simulink model "Spange_Thrust_simulation_4mode"  (R2016a)
settings: Solver=ode3  StartTime=0.0  StopTime=4  RelTol=1e-3
values from neighbouring files (symbols this model uses):
  C = [C1;C2;C3]    [Spange_init.m]
  D = 3.0/100    (= 0.03)    [Spange_init.m]
  eps_c = 5    [Spange_init.m]
  epsilon = 0.5    [Spange_init.m]
  hd = c2d(H1,0.1,'foh')    [Spange_init.m]
  hd2 = c2d(H2,0.01,'zoh')    [Spange_init.m]
  I_s = 0.05    [Spange_init.m]
  k_cc = 1    [Spange_init.m]
  K_omega = 0.3    [Spange_init.m]
  K_q1f = 0.0113    [Spange_init.m]
  K_q1r = K_q1f    (= 0.0113)    [Spange_init.m]
  K_q2f = 0.0117    [Spange_init.m]
  K_q2r = K_q2f    (= 0.0117)    [Spange_init.m]
  K_q3f = 0.0113    [Spange_init.m]
  K_q3r = K_q3f    (= 0.0113)    [Spange_init.m]
  K_T1f = 0.3763    [Spange_init.m]
  K_T1r = K_T1f    (= 0.3763)    [Spange_init.m]
  K_T2f = 0.3901    [Spange_init.m]
  K_T2r = K_T2f    (= 0.3901)    [Spange_init.m]
  K_T3f = 0.3776    [Spange_init.m]
  K_T3r = K_T3f    (= 0.3776)    [Spange_init.m]
  Kp = 0.3    [Spange_init.m]
  Max_Acceleration = 2    [Spange_init.m]
  Max_rotation = 12*sqrt(lambda)    [Spange_init.m]
  Max_thrust = 1.5034    [Spange_init.m]
  Min_thrust = -0.85    [Spange_init.m]
  mode = 4    [Spange_init.m]
  n_c = 5    [Spange_init.m]
  n_max = 64.6    [Spange_init.m]
  p_cc = 0.5    [Spange_init.m]
  Q_f0 = 0.3    [Spange_init.m]
  r_cc = 4    [Spange_init.m]
  Rho = Rho_m    (= 1000)    [Spange_init.m]
  td = [1;0;0]    [Spange_init.m]
  Thruster_control = 1    [Spange_init.m]
  ThrusterPosX = [Thruster.T1(1) Thruster.T2(1) Thruster.T3(1)]    [Spange_init.m]
  ThrusterPosY = [Thruster.T1(2) Thruster.T2(2) Thruster.T3(2)]    [Spange_init.m]
  u_e = [1 0 1 0 0 ... (first row only)    [Spange_init.m]
undefined symbols (not defined in the file or in its folder): Thruster
libraries: simulink_extras x16, simulink x8
(part 2 of 3)

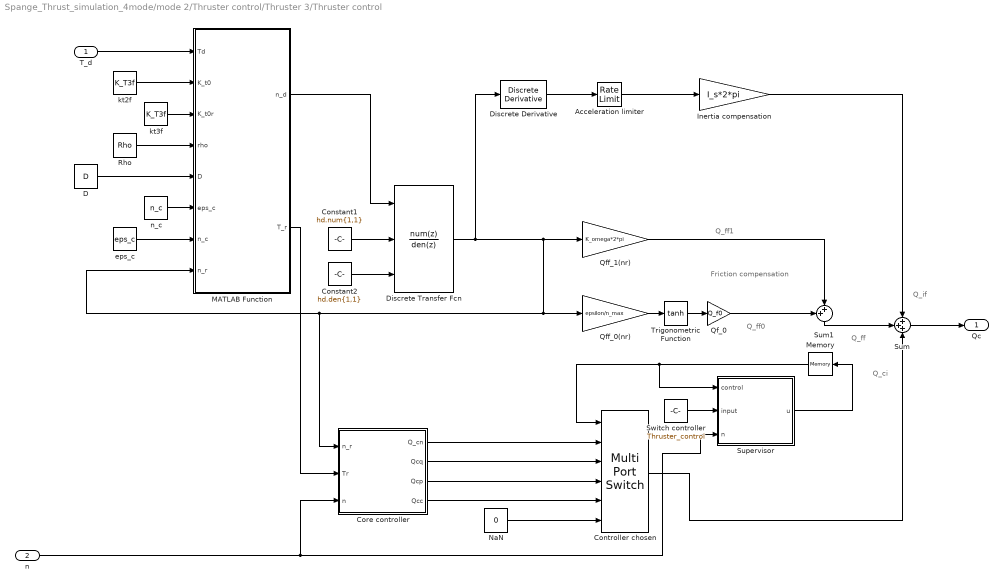
== system Spange_Thrust_simulation_4mode/mode 2/Thruster control/Thruster 3/Thruster control ==
  note: Friction compensation
  note: Q_ff1
  note: Q_ff0
  note: Q_ff
  note: Q_if
  note: Q_ci
  "T_d " : Inport
  n : Inport  Port=2
  Acceleration limiter : RateLimiter  RisingSlewLimit=Max_Acceleration  FallingSlewLimit=-Max_Acceleration  SampleTimeMode=inherited
  Constant1 : Constant  Value=hd.num{1,1}  VectorParams1D=off
  Constant2 : Constant  Value=hd.den{1,1}  VectorParams1D=off
  Controller chosen : MultiPortSwitch  Inputs=5
  Core controller : Subsystem
  D : Constant  Value=D  VectorParams1D=off
  Discrete Transfer Fcn : DiscreteTransferFcn  NumeratorSource=Input port  Numerator=[8.76e-05 0.0003481 8.648e-05]  DenominatorSource=Input port  Denominator=[1 -1.974 0.9746]  SampleTime=0.01  a0EqualsOne=on
      settings: InputPortMap=u0,p1,p3
  Discrete Derivative : simulink/Discrete/Discrete Derivative  gainval=1.0  ICPrevScaledInput=0.0  InputProcessing=Inherited  OutMin=[]  OutMax=[]  OutDataType=fixdt(1, 16)  OutScaling=2^-10  DoSatur=off
  Inertia compensation : Gain  Gain=I_s*2*pi
  MATLAB Function : MATLAB Function  TreatAsAtomicUnit=on
  Memory : Memory  X0=1
  NaN : Constant  Value=0
  Qf_0 : Gain  Gain=Q_f0
  Qff_0(nr) : Gain  Gain=epsilon/n_max
  Qff_1(nr) : Gain  Gain=K_omega*2*pi
  Rho : Constant  Value=Rho  VectorParams1D=off
  Sum : Sum  Inputs=+++
  Sum1 : Sum  Inputs=++|
  Supervisor : MATLAB Function  TreatAsAtomicUnit=on
  Switch controller : Constant  Value=Thruster_control
  Trigonometric Function : Trigonometry  Operator=tanh
  eps_c : Constant  Value=eps_c  VectorParams1D=off
  kt2f : Constant  Value=K_T3f  VectorParams1D=off
  kt3f : Constant  Value=K_T3f  VectorParams1D=off
  n_c : Constant  Value=n_c  VectorParams1D=off
  Qc : Outport
  wires:
  kt3f/1 -> MATLAB Function/3(K_t0r)
  kt2f/1 -> MATLAB Function/2(K_t0)
  Sum/1 -> Qc/1
  Discrete Transfer Fcn/1 -> Qff_1(nr)/1, Qff_0(nr)/1, Core controller/1(n_r), MATLAB Function/8(n_r), Discrete Derivative/1
  Acceleration limiter/1 -> Inertia compensation/1
  n/1 -> Supervisor/3(n), Core controller/3("n ")
  MATLAB Function/1(n_d) -> Discrete Transfer Fcn/1
  Constant2/1 -> Discrete Transfer Fcn/3
  Constant1/1 -> Discrete Transfer Fcn/2
  eps_c/1 -> MATLAB Function/7(n_c)
  n_c/1 -> MATLAB Function/6(eps_c)
  D/1 -> MATLAB Function/5(D)
  Rho/1 -> MATLAB Function/4(rho)
  "T_d "/1 -> MATLAB Function/1(Td)
  Switch controller/1 -> Supervisor/2(input)
  Core controller/2(Qcq) -> Controller chosen/3
  Core controller/3(Qcp) -> Controller chosen/4
  Inertia compensation/1 -> Sum/1
  Controller chosen/1 -> Sum/3
  Qf_0/1 -> Sum1/1
  Qff_1(nr)/1 -> Sum1/2
  Memory/1 -> Controller chosen/1, Supervisor/1(control)
  Supervisor/1(u) -> Memory/1
  NaN/1 -> Controller chosen/6
  Core controller/4(Qcc) -> Controller chosen/5
  Core controller/1(Q_cn) -> Controller chosen/2
  Sum1/1 -> Sum/2
  Trigonometric Function/1 -> Qf_0/1
  Qff_0(nr)/1 -> Trigonometric Function/1
  Discrete Derivative/1 -> Acceleration limiter/1
  MATLAB Function/2(T_r) -> Core controller/2("Tr ")

== system Spange_Thrust_simulation_4mode/mode 3/Thruster control/Thruster 1/Propeller Hydrodynamics ==
  env : Inport
  n : Inport  Port=2
  Actual Force and Torque : MATLAB Function  TreatAsAtomicUnit=on
  D1 : Constant  Value=D
  Kq1 : Constant  Value=K_q1f
  Kqr1 : Constant  Value=K_q1r
  Ktf : Constant  Value=K_T1f
  Ktr : Constant  Value=K_T1r
  Rho1 : Constant  Value=Rho
  eps_c1 : Constant  Value=eps_c
  Ta : Outport
  Qa : Outport  Port=2
  wires:
  eps_c1/1 -> Actual Force and Torque/8(eps_c)
  Kqr1/1 -> Actual Force and Torque/5(Kqr)
  Ktr/1 -> Actual Force and Torque/4(Ktr)
  Actual Force and Torque/1(Ta) -> Ta/1
  Ktf/1 -> Actual Force and Torque/3(Kt)
  env/1 -> Actual Force and Torque/9(env)
  Rho1/1 -> Actual Force and Torque/6(Rho)
  Actual Force and Torque/2(Qa) -> Qa/1
  Kq1/1 -> Actual Force and Torque/2(Kq)
  D1/1 -> Actual Force and Torque/7(D)
  n/1 -> Actual Force and Torque/1(n)

== system Spange_Thrust_simulation_4mode/mode 3/Thruster control/Thruster 1/Shaft dynamics ==
  Qm : Inport
  Qa : Inport  Port=2
  Constant : Constant  Value=0
  Finding rotation speed : Gain  Gain=1/(2*pi*I_s)
  Integrator : Integrator  ExternalReset=either
  K_omega : Gain  Gain=K_omega*2*pi
  Sum : Sum  Inputs=-+-
  n : Outport
  wires:
  Constant/1 -> Integrator/2
  Integrator/1 -> K_omega/1, n/1
  Finding rotation speed/1 -> Integrator/1
  K_omega/1 -> Sum/3
  Qa/1 -> Sum/1
  Sum/1 -> Finding rotation speed/1
  Qm/1 -> Sum/2

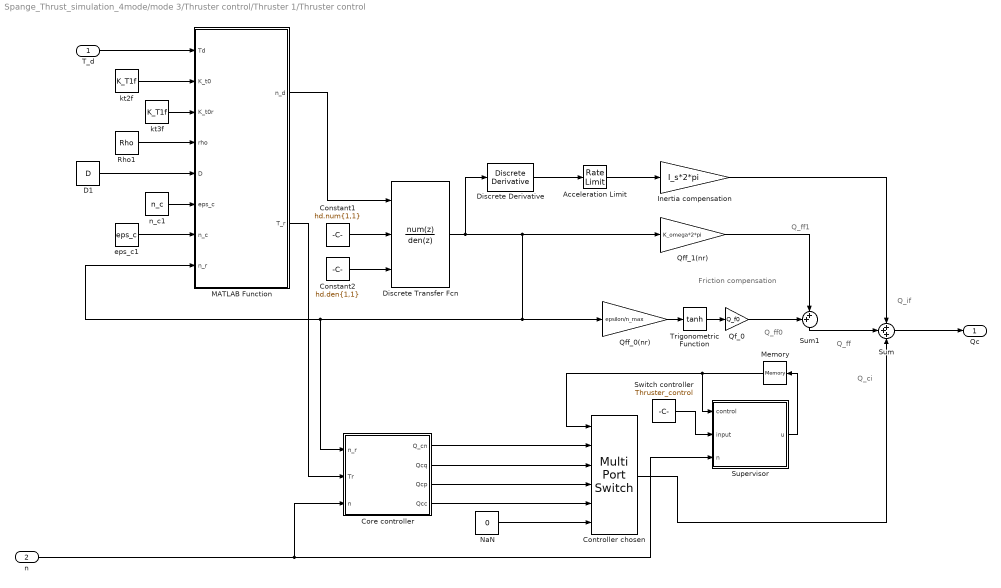
== system Spange_Thrust_simulation_4mode/mode 3/Thruster control/Thruster 1/Thruster control ==
  note: Friction compensation
  note: Q_ff1
  note: Q_ff0
  note: Q_ff
  note: Q_if
  note: Q_ci
  "T_d " : Inport
  n : Inport  Port=2
  Acceleration Limit : RateLimiter  RisingSlewLimit=Max_Acceleration  FallingSlewLimit=-Max_Acceleration  SampleTimeMode=inherited
  Constant1 : Constant  Value=hd.num{1,1}  VectorParams1D=off
  Constant2 : Constant  Value=hd.den{1,1}  VectorParams1D=off
  Controller chosen : MultiPortSwitch  Inputs=5
  Core controller : Subsystem
  D1 : Constant  Value=D  VectorParams1D=off
  Discrete Transfer Fcn : DiscreteTransferFcn  NumeratorSource=Input port  Numerator=[8.76e-05 0.0003481 8.648e-05]  DenominatorSource=Input port  Denominator=[1 -1.974 0.9746]  SampleTime=0.01  a0EqualsOne=on
      settings: InputPortMap=u0,p1,p3
  Discrete Derivative : simulink/Discrete/Discrete Derivative  gainval=1.0  ICPrevScaledInput=0.0  InputProcessing=Inherited  OutMin=[]  OutMax=[]  OutDataType=fixdt(1, 16)  OutScaling=2^-10  DoSatur=off
  Inertia compensation : Gain  Gain=I_s*2*pi
  MATLAB Function : MATLAB Function  TreatAsAtomicUnit=on
  Memory : Memory  X0=1  InheritSampleTime=on
  NaN : Constant  Value=0
  Qf_0 : Gain  Gain=Q_f0
  Qff_0(nr) : Gain  Gain=epsilon/n_max
  Qff_1(nr) : Gain  Gain=K_omega*2*pi
  Rho1 : Constant  Value=Rho  VectorParams1D=off
  Sum : Sum  Inputs=+++
  Sum1 : Sum  Inputs=++|
  Supervisor : MATLAB Function  TreatAsAtomicUnit=on
  Switch controller : Constant  Value=Thruster_control
  Trigonometric Function : Trigonometry  Operator=tanh
  eps_c1 : Constant  Value=eps_c  VectorParams1D=off
  kt2f : Constant  Value=K_T1f  VectorParams1D=off
  kt3f : Constant  Value=K_T1f  VectorParams1D=off
  n_c1 : Constant  Value=n_c  VectorParams1D=off
  Qc : Outport
  wires:
  Sum/1 -> Qc/1
  "T_d "/1 -> MATLAB Function/1(Td)
  Discrete Transfer Fcn/1 -> Discrete Derivative/1, Qff_1(nr)/1, Qff_0(nr)/1, MATLAB Function/8(n_r), Core controller/1(n_r)
  Acceleration Limit/1 -> Inertia compensation/1
  n/1 -> Supervisor/3(n), Core controller/3("n ")
  Inertia compensation/1 -> Sum/1
  Constant2/1 -> Discrete Transfer Fcn/3
  Constant1/1 -> Discrete Transfer Fcn/2
  Sum1/1 -> Sum/2
  Discrete Derivative/1 -> Acceleration Limit/1
  Core controller/1(Q_cn) -> Controller chosen/2
  Core controller/4(Qcc) -> Controller chosen/5
  Core controller/3(Qcp) -> Controller chosen/4
  Core controller/2(Qcq) -> Controller chosen/3
  Controller chosen/1 -> Sum/3
  Switch controller/1 -> Supervisor/2(input)
  Qf_0/1 -> Sum1/1
  Qff_1(nr)/1 -> Sum1/2
  Memory/1 -> Supervisor/1(control), Controller chosen/1
  Supervisor/1(u) -> Memory/1
  NaN/1 -> Controller chosen/6
  Trigonometric Function/1 -> Qf_0/1
  Qff_0(nr)/1 -> Trigonometric Function/1
  MATLAB Function/1(n_d) -> Discrete Transfer Fcn/1
  MATLAB Function/2(T_r) -> Core controller/2("Tr ")
  kt2f/1 -> MATLAB Function/2(K_t0)
  eps_c1/1 -> MATLAB Function/7(n_c)
  D1/1 -> MATLAB Function/5(D)
  Rho1/1 -> MATLAB Function/4(rho)
  kt3f/1 -> MATLAB Function/3(K_t0r)
  n_c1/1 -> MATLAB Function/6(eps_c)

== system Spange_Thrust_simulation_4mode/mode 3/Thruster control/Thruster 2/Propeller Hydrodynamics ==
  env : Inport
  n : Inport  Port=2
  Actual Force and Torque : MATLAB Function  TreatAsAtomicUnit=on
  D1 : Constant  Value=D
  Kq1 : Constant  Value=K_q2f
  Kqr1 : Constant  Value=K_q2r
  Ktf : Constant  Value=K_T2f
  Ktr : Constant  Value=K_T2r
  Rho1 : Constant  Value=Rho
  eps_c1 : Constant  Value=eps_c
  Ta : Outport
  Qa : Outport  Port=2
  wires:
  eps_c1/1 -> Actual Force and Torque/8(eps_c)
  Kqr1/1 -> Actual Force and Torque/5(Kqr)
  Ktr/1 -> Actual Force and Torque/4(Ktr)
  Actual Force and Torque/1(Ta) -> Ta/1
  Ktf/1 -> Actual Force and Torque/3(Kt)
  env/1 -> Actual Force and Torque/9(env)
  Rho1/1 -> Actual Force and Torque/6(Rho)
  Actual Force and Torque/2(Qa) -> Qa/1
  Kq1/1 -> Actual Force and Torque/2(Kq)
  D1/1 -> Actual Force and Torque/7(D)
  n/1 -> Actual Force and Torque/1(n)

== system Spange_Thrust_simulation_4mode/mode 3/Thruster control/Thruster 2/Shaft dynamics ==
  Qm : Inport
  Qa : Inport  Port=2
  Constant : Constant  Value=0
  Finding rotation speed : Gain  Gain=1/(2*pi*I_s)
  Integrator : Integrator  ExternalReset=either
  K_omega : Gain  Gain=K_omega*2*pi
  Sum : Sum  Inputs=-+-
  n : Outport
  wires:
  Constant/1 -> Integrator/2
  Integrator/1 -> n/1, K_omega/1
  Finding rotation speed/1 -> Integrator/1
  K_omega/1 -> Sum/3
  Qa/1 -> Sum/1
  Sum/1 -> Finding rotation speed/1
  Qm/1 -> Sum/2

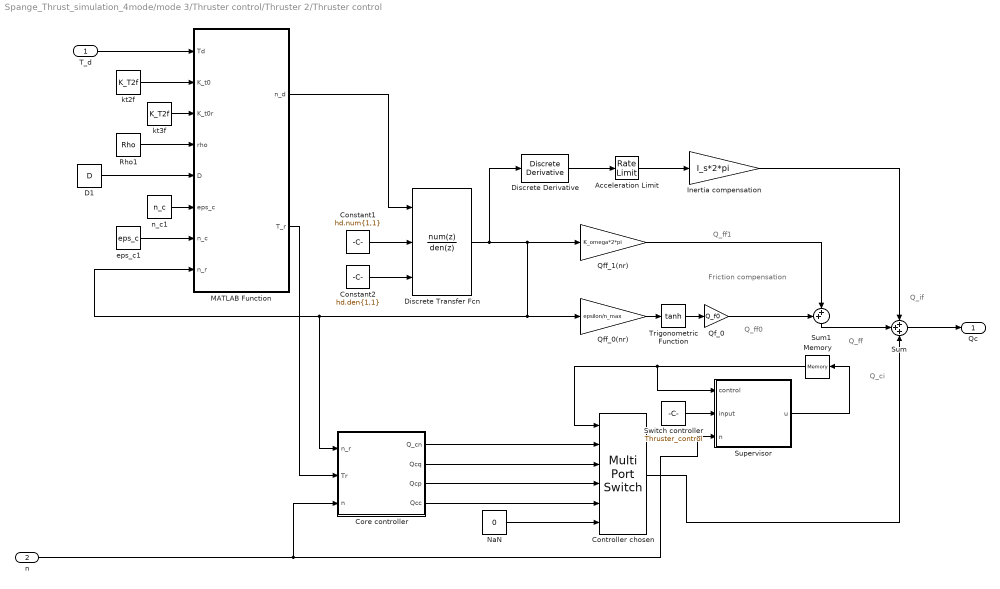
== system Spange_Thrust_simulation_4mode/mode 3/Thruster control/Thruster 2/Thruster control ==
  note: Friction compensation
  note: Q_ff1
  note: Q_ff0
  note: Q_ff
  note: Q_if
  note: Q_ci
  "T_d " : Inport
  n : Inport  Port=2
  Acceleration Limit : RateLimiter  RisingSlewLimit=Max_Acceleration  FallingSlewLimit=-Max_Acceleration  SampleTimeMode=inherited
  Constant1 : Constant  Value=hd.num{1,1}  VectorParams1D=off
  Constant2 : Constant  Value=hd.den{1,1}  VectorParams1D=off
  Controller chosen : MultiPortSwitch  Inputs=5
  Core controller : Subsystem
  D1 : Constant  Value=D  VectorParams1D=off
  Discrete Transfer Fcn : DiscreteTransferFcn  NumeratorSource=Input port  Numerator=[8.76e-05 0.0003481 8.648e-05]  DenominatorSource=Input port  Denominator=[1 -1.974 0.9746]  SampleTime=0.01  a0EqualsOne=on
      settings: InputPortMap=u0,p1,p3
  Discrete Derivative : simulink/Discrete/Discrete Derivative  gainval=1.0  ICPrevScaledInput=0.0  InputProcessing=Inherited  OutMin=[]  OutMax=[]  OutDataType=fixdt(1, 16)  OutScaling=2^-10  DoSatur=off
  Inertia compensation : Gain  Gain=I_s*2*pi
  MATLAB Function : MATLAB Function  TreatAsAtomicUnit=on
  Memory : Memory  X0=1
  NaN : Constant  Value=0
  Qf_0 : Gain  Gain=Q_f0
  Qff_0(nr) : Gain  Gain=epsilon/n_max
  Qff_1(nr) : Gain  Gain=K_omega*2*pi
  Rho1 : Constant  Value=Rho  VectorParams1D=off
  Sum : Sum  Inputs=+++
  Sum1 : Sum  Inputs=++|
  Supervisor : MATLAB Function  TreatAsAtomicUnit=on
  Switch controller : Constant  Value=Thruster_control
  Trigonometric Function : Trigonometry  Operator=tanh
  eps_c1 : Constant  Value=eps_c  VectorParams1D=off
  kt2f : Constant  Value=K_T2f  VectorParams1D=off
  kt3f : Constant  Value=K_T2f  VectorParams1D=off
  n_c1 : Constant  Value=n_c  VectorParams1D=off
  Qc : Outport
  wires:
  Sum/1 -> Qc/1
  Discrete Transfer Fcn/1 -> Qff_1(nr)/1, Core controller/1(n_r), MATLAB Function/8(n_r), Qff_0(nr)/1, Discrete Derivative/1
  Acceleration Limit/1 -> Inertia compensation/1
  n/1 -> Supervisor/3(n), Core controller/3("n ")
  Discrete Derivative/1 -> Acceleration Limit/1
  MATLAB Function/1(n_d) -> Discrete Transfer Fcn/1
  Constant2/1 -> Discrete Transfer Fcn/3
  Constant1/1 -> Discrete Transfer Fcn/2
  "T_d "/1 -> MATLAB Function/1(Td)
  Switch controller/1 -> Supervisor/2(input)
  Core controller/2(Qcq) -> Controller chosen/3
  Core controller/3(Qcp) -> Controller chosen/4
  Inertia compensation/1 -> Sum/1
  Controller chosen/1 -> Sum/3
  Qf_0/1 -> Sum1/1
  Qff_1(nr)/1 -> Sum1/2
  Memory/1 -> Controller chosen/1, Supervisor/1(control)
  Supervisor/1(u) -> Memory/1
  NaN/1 -> Controller chosen/6
  Core controller/4(Qcc) -> Controller chosen/5
  Core controller/1(Q_cn) -> Controller chosen/2
  Sum1/1 -> Sum/2
  Trigonometric Function/1 -> Qf_0/1
  Qff_0(nr)/1 -> Trigonometric Function/1
  MATLAB Function/2(T_r) -> Core controller/2("Tr ")
  kt2f/1 -> MATLAB Function/2(K_t0)
  eps_c1/1 -> MATLAB Function/7(n_c)
  D1/1 -> MATLAB Function/5(D)
  Rho1/1 -> MATLAB Function/4(rho)
  kt3f/1 -> MATLAB Function/3(K_t0r)
  n_c1/1 -> MATLAB Function/6(eps_c)

== system Spange_Thrust_simulation_4mode/mode 4/Thruster control/Thruster 1/Propeller Hydrodynamics ==
  env : Inport
  n : Inport  Port=2
  Actual Force and Torque : MATLAB Function  TreatAsAtomicUnit=on
  D1 : Constant  Value=D
  Kq1 : Constant  Value=K_q1f
  Kqr1 : Constant  Value=K_q1r
  Ktf : Constant  Value=K_T1f
  Ktr : Constant  Value=K_T1r
  Rho1 : Constant  Value=Rho
  eps_c1 : Constant  Value=eps_c
  Ta : Outport
  Qa : Outport  Port=2
  wires:
  eps_c1/1 -> Actual Force and Torque/8(eps_c)
  Kqr1/1 -> Actual Force and Torque/5(Kqr)
  Ktr/1 -> Actual Force and Torque/4(Ktr)
  Actual Force and Torque/1(Ta) -> Ta/1
  Ktf/1 -> Actual Force and Torque/3(Kt)
  env/1 -> Actual Force and Torque/9(env)
  Rho1/1 -> Actual Force and Torque/6(Rho)
  Actual Force and Torque/2(Qa) -> Qa/1
  Kq1/1 -> Actual Force and Torque/2(Kq)
  D1/1 -> Actual Force and Torque/7(D)
  n/1 -> Actual Force and Torque/1(n)

== system Spange_Thrust_simulation_4mode/mode 4/Thruster control/Thruster 1/Shaft dynamics ==
  Qm : Inport
  Qa : Inport  Port=2
  Constant : Constant  Value=0
  Finding rotation speed : Gain  Gain=1/(2*pi*I_s)
  Integrator : Integrator  ExternalReset=either
  K_omega : Gain  Gain=K_omega*2*pi
  Sum : Sum  Inputs=-+-
  n : Outport
  wires:
  Constant/1 -> Integrator/2
  Integrator/1 -> K_omega/1, n/1
  Finding rotation speed/1 -> Integrator/1
  K_omega/1 -> Sum/3
  Qa/1 -> Sum/1
  Sum/1 -> Finding rotation speed/1
  Qm/1 -> Sum/2

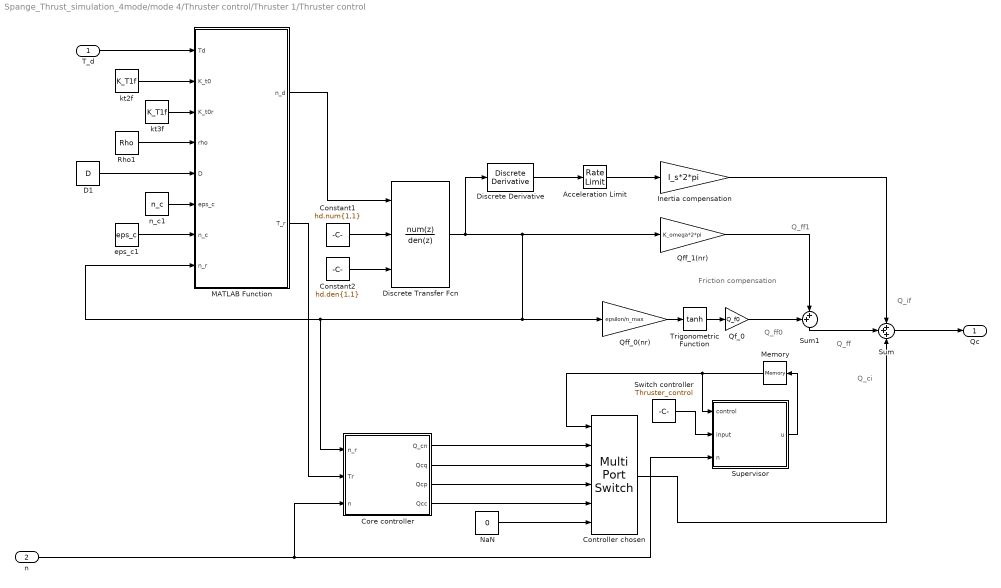
== system Spange_Thrust_simulation_4mode/mode 4/Thruster control/Thruster 1/Thruster control ==
  note: Friction compensation
  note: Q_ff1
  note: Q_ff0
  note: Q_ff
  note: Q_if
  note: Q_ci
  "T_d " : Inport
  n : Inport  Port=2
  Acceleration Limit : RateLimiter  RisingSlewLimit=Max_Acceleration  FallingSlewLimit=-Max_Acceleration  SampleTimeMode=inherited
  Constant1 : Constant  Value=hd.num{1,1}  VectorParams1D=off
  Constant2 : Constant  Value=hd.den{1,1}  VectorParams1D=off
  Controller chosen : MultiPortSwitch  Inputs=5
  Core controller : Subsystem
  D1 : Constant  Value=D  VectorParams1D=off
  Discrete Transfer Fcn : DiscreteTransferFcn  NumeratorSource=Input port  Numerator=[8.76e-05 0.0003481 8.648e-05]  DenominatorSource=Input port  Denominator=[1 -1.974 0.9746]  SampleTime=0.01  a0EqualsOne=on
      settings: InputPortMap=u0,p1,p3
  Discrete Derivative : simulink/Discrete/Discrete Derivative  gainval=1.0  ICPrevScaledInput=0.0  InputProcessing=Inherited  OutMin=[]  OutMax=[]  OutDataType=fixdt(1, 16)  OutScaling=2^-10  DoSatur=off
  Inertia compensation : Gain  Gain=I_s*2*pi
  MATLAB Function : MATLAB Function  TreatAsAtomicUnit=on
  Memory : Memory  X0=1  InheritSampleTime=on
  NaN : Constant  Value=0
  Qf_0 : Gain  Gain=Q_f0
  Qff_0(nr) : Gain  Gain=epsilon/n_max
  Qff_1(nr) : Gain  Gain=K_omega*2*pi
  Rho1 : Constant  Value=Rho  VectorParams1D=off
  Sum : Sum  Inputs=+++
  Sum1 : Sum  Inputs=++|
  Supervisor : MATLAB Function  TreatAsAtomicUnit=on
  Switch controller : Constant  Value=Thruster_control
  Trigonometric Function : Trigonometry  Operator=tanh
  eps_c1 : Constant  Value=eps_c  VectorParams1D=off
  kt2f : Constant  Value=K_T1f  VectorParams1D=off
  kt3f : Constant  Value=K_T1f  VectorParams1D=off
  n_c1 : Constant  Value=n_c  VectorParams1D=off
  Qc : Outport
  wires:
  Sum/1 -> Qc/1
  "T_d "/1 -> MATLAB Function/1(Td)
  Discrete Transfer Fcn/1 -> Discrete Derivative/1, Qff_1(nr)/1, Qff_0(nr)/1, MATLAB Function/8(n_r), Core controller/1(n_r)
  Acceleration Limit/1 -> Inertia compensation/1
  n/1 -> Supervisor/3(n), Core controller/3("n ")
  Inertia compensation/1 -> Sum/1
  Constant2/1 -> Discrete Transfer Fcn/3
  Constant1/1 -> Discrete Transfer Fcn/2
  Sum1/1 -> Sum/2
  Discrete Derivative/1 -> Acceleration Limit/1
  Core controller/1(Q_cn) -> Controller chosen/2
  Core controller/4(Qcc) -> Controller chosen/5
  Core controller/3(Qcp) -> Controller chosen/4
  Core controller/2(Qcq) -> Controller chosen/3
  Controller chosen/1 -> Sum/3
  Switch controller/1 -> Supervisor/2(input)
  Qf_0/1 -> Sum1/1
  Qff_1(nr)/1 -> Sum1/2
  Memory/1 -> Supervisor/1(control), Controller chosen/1
  Supervisor/1(u) -> Memory/1
  NaN/1 -> Controller chosen/6
  Trigonometric Function/1 -> Qf_0/1
  Qff_0(nr)/1 -> Trigonometric Function/1
  MATLAB Function/1(n_d) -> Discrete Transfer Fcn/1
  MATLAB Function/2(T_r) -> Core controller/2("Tr ")
  kt2f/1 -> MATLAB Function/2(K_t0)
  eps_c1/1 -> MATLAB Function/7(n_c)
  D1/1 -> MATLAB Function/5(D)
  Rho1/1 -> MATLAB Function/4(rho)
  kt3f/1 -> MATLAB Function/3(K_t0r)
  n_c1/1 -> MATLAB Function/6(eps_c)

== system Spange_Thrust_simulation_4mode/mode 4/Thruster control/Thruster 2/Propeller Hydrodynamics ==
  env : Inport
  n : Inport  Port=2
  Actual Force and Torque : MATLAB Function  TreatAsAtomicUnit=on
  D1 : Constant  Value=D
  Kq1 : Constant  Value=K_q2f
  Kqr1 : Constant  Value=K_q2r
  Ktf : Constant  Value=K_T2f
  Ktr : Constant  Value=K_T2r
  Rho1 : Constant  Value=Rho
  eps_c1 : Constant  Value=eps_c
  Ta : Outport
  Qa : Outport  Port=2
  wires:
  eps_c1/1 -> Actual Force and Torque/8(eps_c)
  Kqr1/1 -> Actual Force and Torque/5(Kqr)
  Ktr/1 -> Actual Force and Torque/4(Ktr)
  Actual Force and Torque/1(Ta) -> Ta/1
  Ktf/1 -> Actual Force and Torque/3(Kt)
  env/1 -> Actual Force and Torque/9(env)
  Rho1/1 -> Actual Force and Torque/6(Rho)
  Actual Force and Torque/2(Qa) -> Qa/1
  Kq1/1 -> Actual Force and Torque/2(Kq)
  D1/1 -> Actual Force and Torque/7(D)
  n/1 -> Actual Force and Torque/1(n)

== system Spange_Thrust_simulation_4mode/mode 4/Thruster control/Thruster 2/Shaft dynamics ==
  Qm : Inport
  Qa : Inport  Port=2
  Constant : Constant  Value=0
  Finding rotation speed : Gain  Gain=1/(2*pi*I_s)
  Integrator : Integrator  ExternalReset=either
  K_omega : Gain  Gain=K_omega*2*pi
  Sum : Sum  Inputs=-+-
  n : Outport
  wires:
  Constant/1 -> Integrator/2
  Integrator/1 -> n/1, K_omega/1
  Finding rotation speed/1 -> Integrator/1
  K_omega/1 -> Sum/3
  Qa/1 -> Sum/1
  Sum/1 -> Finding rotation speed/1
  Qm/1 -> Sum/2

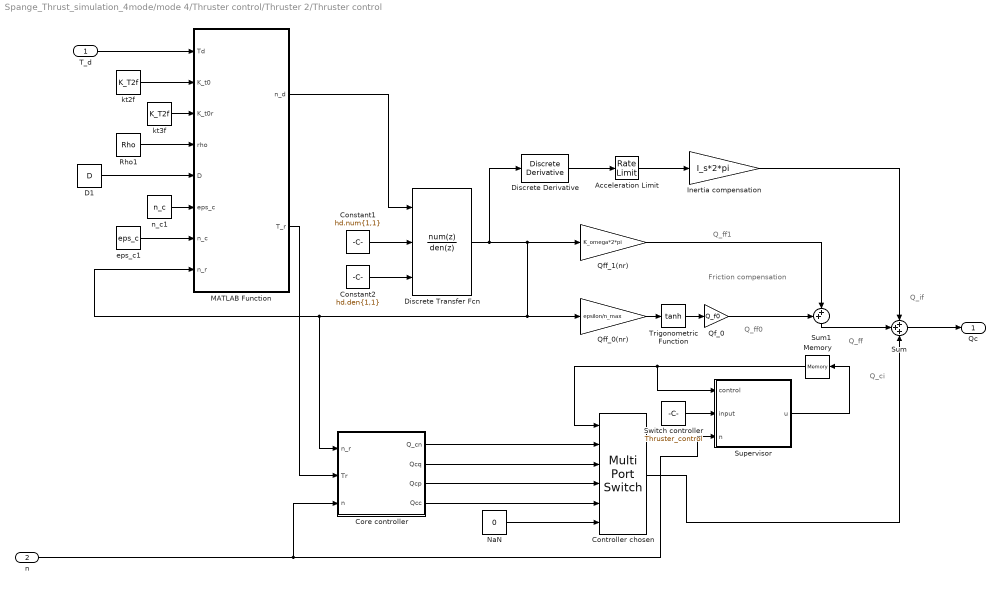
== system Spange_Thrust_simulation_4mode/mode 4/Thruster control/Thruster 2/Thruster control ==
  note: Friction compensation
  note: Q_ff1
  note: Q_ff0
  note: Q_ff
  note: Q_if
  note: Q_ci
  "T_d " : Inport
  n : Inport  Port=2
  Acceleration Limit : RateLimiter  RisingSlewLimit=Max_Acceleration  FallingSlewLimit=-Max_Acceleration  SampleTimeMode=inherited
  Constant1 : Constant  Value=hd.num{1,1}  VectorParams1D=off
  Constant2 : Constant  Value=hd.den{1,1}  VectorParams1D=off
  Controller chosen : MultiPortSwitch  Inputs=5
  Core controller : Subsystem
  D1 : Constant  Value=D  VectorParams1D=off
  Discrete Transfer Fcn : DiscreteTransferFcn  NumeratorSource=Input port  Numerator=[8.76e-05 0.0003481 8.648e-05]  DenominatorSource=Input port  Denominator=[1 -1.974 0.9746]  SampleTime=0.01  a0EqualsOne=on
      settings: InputPortMap=u0,p1,p3
  Discrete Derivative : simulink/Discrete/Discrete Derivative  gainval=1.0  ICPrevScaledInput=0.0  InputProcessing=Inherited  OutMin=[]  OutMax=[]  OutDataType=fixdt(1, 16)  OutScaling=2^-10  DoSatur=off
  Inertia compensation : Gain  Gain=I_s*2*pi
  MATLAB Function : MATLAB Function  TreatAsAtomicUnit=on
  Memory : Memory  X0=1
  NaN : Constant  Value=0
  Qf_0 : Gain  Gain=Q_f0
  Qff_0(nr) : Gain  Gain=epsilon/n_max
  Qff_1(nr) : Gain  Gain=K_omega*2*pi
  Rho1 : Constant  Value=Rho  VectorParams1D=off
  Sum : Sum  Inputs=+++
  Sum1 : Sum  Inputs=++|
  Supervisor : MATLAB Function  TreatAsAtomicUnit=on
  Switch controller : Constant  Value=Thruster_control
  Trigonometric Function : Trigonometry  Operator=tanh
  eps_c1 : Constant  Value=eps_c  VectorParams1D=off
  kt2f : Constant  Value=K_T2f  VectorParams1D=off
  kt3f : Constant  Value=K_T2f  VectorParams1D=off
  n_c1 : Constant  Value=n_c  VectorParams1D=off
  Qc : Outport
  wires:
  Sum/1 -> Qc/1
  Discrete Transfer Fcn/1 -> Qff_1(nr)/1, Core controller/1(n_r), MATLAB Function/8(n_r), Qff_0(nr)/1, Discrete Derivative/1
  Acceleration Limit/1 -> Inertia compensation/1
  n/1 -> Supervisor/3(n), Core controller/3("n ")
  Discrete Derivative/1 -> Acceleration Limit/1
  MATLAB Function/1(n_d) -> Discrete Transfer Fcn/1
  Constant2/1 -> Discrete Transfer Fcn/3
  Constant1/1 -> Discrete Transfer Fcn/2
  "T_d "/1 -> MATLAB Function/1(Td)
  Switch controller/1 -> Supervisor/2(input)
  Core controller/2(Qcq) -> Controller chosen/3
  Core controller/3(Qcp) -> Controller chosen/4
  Inertia compensation/1 -> Sum/1
  Controller chosen/1 -> Sum/3
  Qf_0/1 -> Sum1/1
  Qff_1(nr)/1 -> Sum1/2
  Memory/1 -> Controller chosen/1, Supervisor/1(control)
  Supervisor/1(u) -> Memory/1
  NaN/1 -> Controller chosen/6
  Core controller/4(Qcc) -> Controller chosen/5
  Core controller/1(Q_cn) -> Controller chosen/2
  Sum1/1 -> Sum/2
  Trigonometric Function/1 -> Qf_0/1
  Qff_0(nr)/1 -> Trigonometric Function/1
  MATLAB Function/2(T_r) -> Core controller/2("Tr ")
  kt2f/1 -> MATLAB Function/2(K_t0)
  eps_c1/1 -> MATLAB Function/7(n_c)
  D1/1 -> MATLAB Function/5(D)
  Rho1/1 -> MATLAB Function/4(rho)
  kt3f/1 -> MATLAB Function/3(K_t0r)
  n_c1/1 -> MATLAB Function/6(eps_c)

== system Spange_Thrust_simulation_4mode/mode 4/Thruster control/Thruster 3/Propeller Hydrodynamics ==
  env : Inport
  n : Inport  Port=2
  Actual Force and Torque : MATLAB Function  TreatAsAtomicUnit=on
  D : Constant  Value=D
  Kq : Constant  Value=K_q3f
  Kqr : Constant  Value=K_q3r
  Ktf : Constant  Value=K_T3f
  Ktr : Constant  Value=K_T3r
  Rho : Constant  Value=Rho
  eps_c : Constant  Value=eps_c
  Ta : Outport
  Qa : Outport  Port=2
  wires:
  eps_c/1 -> Actual Force and Torque/8(eps_c)
  Kqr/1 -> Actual Force and Torque/5(Kqr)
  Ktr/1 -> Actual Force and Torque/4(Ktr)
  Actual Force and Torque/1(Ta) -> Ta/1
  Ktf/1 -> Actual Force and Torque/3(Kt)
  env/1 -> Actual Force and Torque/9(env)
  Rho/1 -> Actual Force and Torque/6(Rho)
  Actual Force and Torque/2(Qa) -> Qa/1
  Kq/1 -> Actual Force and Torque/2(Kq)
  D/1 -> Actual Force and Torque/7(D)
  n/1 -> Actual Force and Torque/1(n)

== system Spange_Thrust_simulation_4mode/mode 4/Thruster control/Thruster 3/Shaft dynamics ==
  Qm : Inport
  Qa : Inport  Port=2
  Constant : Constant  Value=0
  Finding rotation speed : Gain  Gain=1/(2*pi*I_s)
  Integrator : Integrator  ExternalReset=either
  K_omega : Gain  Gain=K_omega*2*pi
  Sum : Sum  Inputs=-+-
  n : Outport
  wires:
  Constant/1 -> Integrator/2
  Integrator/1 -> K_omega/1, n/1
  Finding rotation speed/1 -> Integrator/1
  K_omega/1 -> Sum/3
  Qa/1 -> Sum/1
  Sum/1 -> Finding rotation speed/1
  Qm/1 -> Sum/2

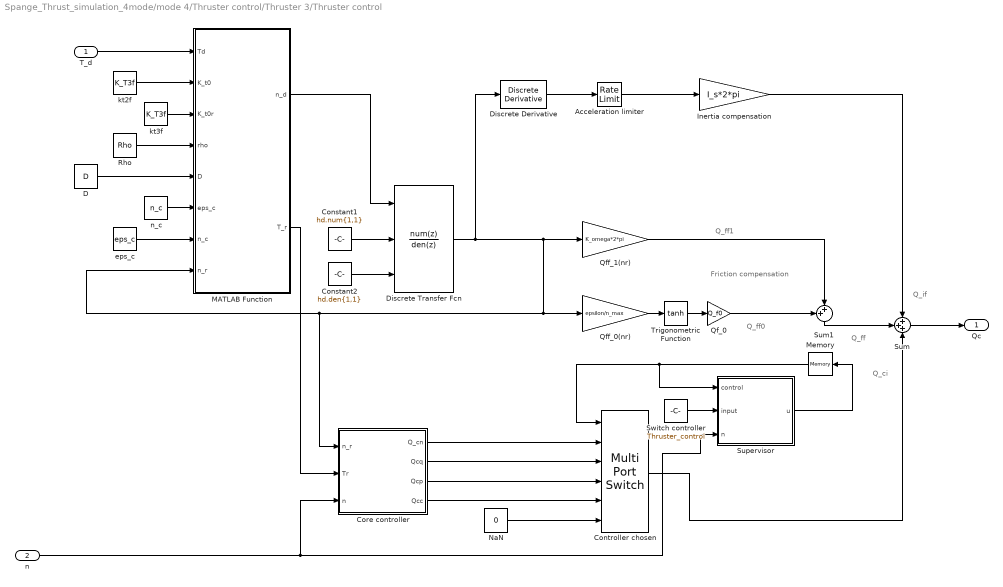
== system Spange_Thrust_simulation_4mode/mode 4/Thruster control/Thruster 3/Thruster control ==
  note: Friction compensation
  note: Q_ff1
  note: Q_ff0
  note: Q_ff
  note: Q_if
  note: Q_ci
  "T_d " : Inport
  n : Inport  Port=2
  Acceleration limiter : RateLimiter  RisingSlewLimit=Max_Acceleration  FallingSlewLimit=-Max_Acceleration  SampleTimeMode=inherited
  Constant1 : Constant  Value=hd.num{1,1}  VectorParams1D=off
  Constant2 : Constant  Value=hd.den{1,1}  VectorParams1D=off
  Controller chosen : MultiPortSwitch  Inputs=5
  Core controller : Subsystem
  D : Constant  Value=D  VectorParams1D=off
  Discrete Transfer Fcn : DiscreteTransferFcn  NumeratorSource=Input port  Numerator=[8.76e-05 0.0003481 8.648e-05]  DenominatorSource=Input port  Denominator=[1 -1.974 0.9746]  SampleTime=0.01  a0EqualsOne=on
      settings: InputPortMap=u0,p1,p3
  Discrete Derivative : simulink/Discrete/Discrete Derivative  gainval=1.0  ICPrevScaledInput=0.0  InputProcessing=Inherited  OutMin=[]  OutMax=[]  OutDataType=fixdt(1, 16)  OutScaling=2^-10  DoSatur=off
  Inertia compensation : Gain  Gain=I_s*2*pi
  MATLAB Function : MATLAB Function  TreatAsAtomicUnit=on
  Memory : Memory  X0=1
  NaN : Constant  Value=0
  Qf_0 : Gain  Gain=Q_f0
  Qff_0(nr) : Gain  Gain=epsilon/n_max
  Qff_1(nr) : Gain  Gain=K_omega*2*pi
  Rho : Constant  Value=Rho  VectorParams1D=off
  Sum : Sum  Inputs=+++
  Sum1 : Sum  Inputs=++|
  Supervisor : MATLAB Function  TreatAsAtomicUnit=on
  Switch controller : Constant  Value=Thruster_control
  Trigonometric Function : Trigonometry  Operator=tanh
  eps_c : Constant  Value=eps_c  VectorParams1D=off
  kt2f : Constant  Value=K_T3f  VectorParams1D=off
  kt3f : Constant  Value=K_T3f  VectorParams1D=off
  n_c : Constant  Value=n_c  VectorParams1D=off
  Qc : Outport
  wires:
  kt3f/1 -> MATLAB Function/3(K_t0r)
  kt2f/1 -> MATLAB Function/2(K_t0)
  Sum/1 -> Qc/1
  Discrete Transfer Fcn/1 -> Qff_1(nr)/1, Qff_0(nr)/1, Core controller/1(n_r), MATLAB Function/8(n_r), Discrete Derivative/1
  Acceleration limiter/1 -> Inertia compensation/1
  n/1 -> Supervisor/3(n), Core controller/3("n ")
  MATLAB Function/1(n_d) -> Discrete Transfer Fcn/1
  Constant2/1 -> Discrete Transfer Fcn/3
  Constant1/1 -> Discrete Transfer Fcn/2
  eps_c/1 -> MATLAB Function/7(n_c)
  n_c/1 -> MATLAB Function/6(eps_c)
  D/1 -> MATLAB Function/5(D)
  Rho/1 -> MATLAB Function/4(rho)
  "T_d "/1 -> MATLAB Function/1(Td)
  Switch controller/1 -> Supervisor/2(input)
  Core controller/2(Qcq) -> Controller chosen/3
  Core controller/3(Qcp) -> Controller chosen/4
  Inertia compensation/1 -> Sum/1
  Controller chosen/1 -> Sum/3
  Qf_0/1 -> Sum1/1
  Qff_1(nr)/1 -> Sum1/2
  Memory/1 -> Controller chosen/1, Supervisor/1(control)
  Supervisor/1(u) -> Memory/1
  NaN/1 -> Controller chosen/6
  Core controller/4(Qcc) -> Controller chosen/5
  Core controller/1(Q_cn) -> Controller chosen/2
  Sum1/1 -> Sum/2
  Trigonometric Function/1 -> Qf_0/1
  Qff_0(nr)/1 -> Trigonometric Function/1
  Discrete Derivative/1 -> Acceleration limiter/1
  MATLAB Function/2(T_r) -> Core controller/2("Tr ")

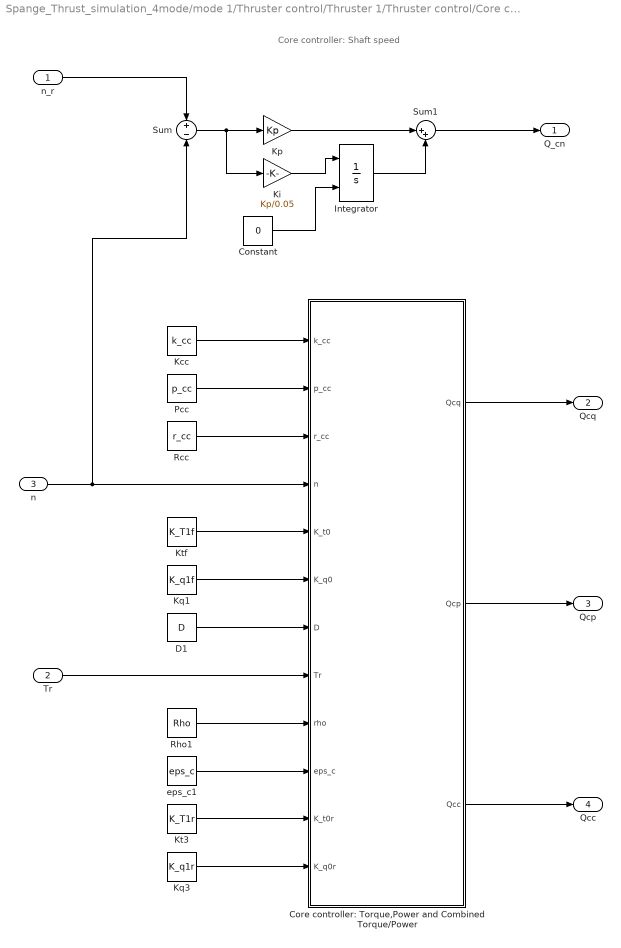
== system Spange_Thrust_simulation_4mode/mode 1/Thruster control/Thruster 1/Thruster control/Core controller ==
  note: Core controller: Shaft speed
  n_r : Inport
  "Tr " : Inport  Port=2
  "n " : Inport  Port=3
  Constant : Constant  Value=0
  Core controller: Torque,Power and Combined Torque/Power : MATLAB Function  TreatAsAtomicUnit=on
  D1 : Constant  Value=D
  Integrator : Integrator  ExternalReset=either
  Kcc : Constant  Value=k_cc
  Ki : Gain  Gain=Kp/0.05
  Kp : Gain  Gain=Kp
  Kq1 : Constant  Value=K_q1f
  "Kq3 " : Constant  Value=K_q1r
  Kt3 : Constant  Value=K_T1r
  Ktf : Constant  Value=K_T1f
  Pcc : Constant  Value=p_cc
  Rcc : Constant  Value=r_cc
  Rho1 : Constant  Value=Rho
  Sum : Sum  Inputs=+|-
  Sum1 : Sum  Inputs=|++
  eps_c1 : Constant  Value=eps_c
  Q_cn : Outport
  Qcq : Outport  Port=2
  Qcp : Outport  Port=3
  Qcc : Outport  Port=4
  wires:
  "Kq3 "/1 -> Core controller: Torque,Power and Combined Torque/Power/12(K_q0r)
  Kq1/1 -> Core controller: Torque,Power and Combined Torque/Power/6(K_q0)
  Kt3/1 -> Core controller: Torque,Power and Combined Torque/Power/11(K_t0r)
  eps_c1/1 -> Core controller: Torque,Power and Combined Torque/Power/10(eps_c)
  Constant/1 -> Integrator/2
  Sum/1 -> Kp/1, Ki/1
  Sum1/1 -> Q_cn/1
  Integrator/1 -> Sum1/2
  Kp/1 -> Sum1/1
  Ki/1 -> Integrator/1
  n_r/1 -> Sum/1
  Core controller: Torque,Power and Combined Torque/Power/1(Qcq) -> Qcq/1
  Core controller: Torque,Power and Combined Torque/Power/2(Qcp) -> Qcp/1
  "Tr "/1 -> Core controller: Torque,Power and Combined Torque/Power/8(Tr)
  "n "/1 -> Core controller: Torque,Power and Combined Torque/Power/4(n), Sum/2
  Rho1/1 -> Core controller: Torque,Power and Combined Torque/Power/9(rho)
  D1/1 -> Core controller: Torque,Power and Combined Torque/Power/7(D)
  Ktf/1 -> Core controller: Torque,Power and Combined Torque/Power/5(K_t0)
  Core controller: Torque,Power and Combined Torque/Power/3(Qcc) -> Qcc/1
  Rcc/1 -> Core controller: Torque,Power and Combined Torque/Power/3(r_cc)
  Pcc/1 -> Core controller: Torque,Power and Combined Torque/Power/2(p_cc)
  Kcc/1 -> Core controller: Torque,Power and Combined Torque/Power/1(k_cc)

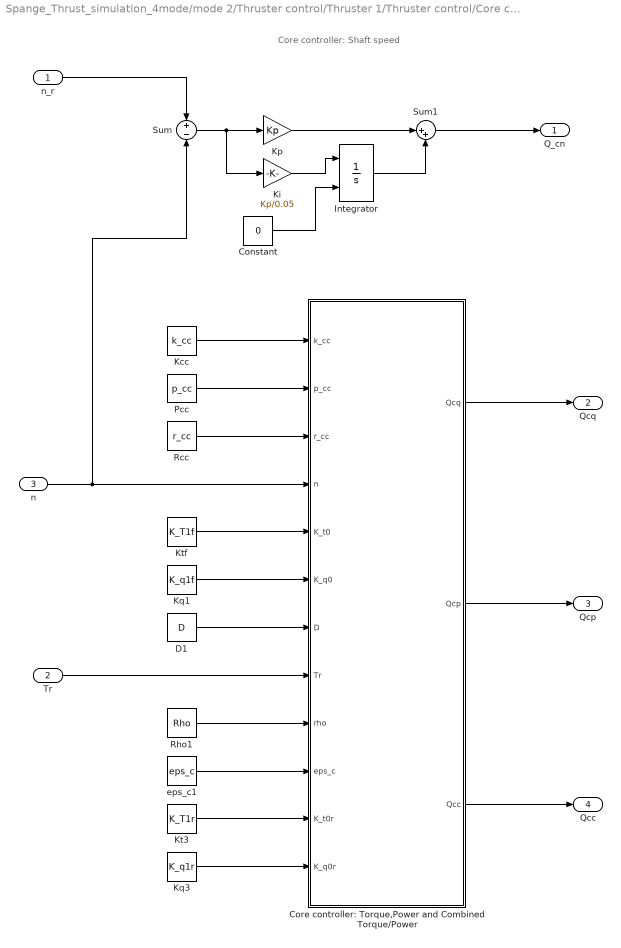
== system Spange_Thrust_simulation_4mode/mode 2/Thruster control/Thruster 1/Thruster control/Core controller ==
  note: Core controller: Shaft speed
  n_r : Inport
  "Tr " : Inport  Port=2
  "n " : Inport  Port=3
  Constant : Constant  Value=0
  Core controller: Torque,Power and Combined Torque/Power : MATLAB Function  TreatAsAtomicUnit=on
  D1 : Constant  Value=D
  Integrator : Integrator  ExternalReset=either
  Kcc : Constant  Value=k_cc
  Ki : Gain  Gain=Kp/0.05
  Kp : Gain  Gain=Kp
  Kq1 : Constant  Value=K_q1f
  "Kq3 " : Constant  Value=K_q1r
  Kt3 : Constant  Value=K_T1r
  Ktf : Constant  Value=K_T1f
  Pcc : Constant  Value=p_cc
  Rcc : Constant  Value=r_cc
  Rho1 : Constant  Value=Rho
  Sum : Sum  Inputs=+|-
  Sum1 : Sum  Inputs=|++
  eps_c1 : Constant  Value=eps_c
  Q_cn : Outport
  Qcq : Outport  Port=2
  Qcp : Outport  Port=3
  Qcc : Outport  Port=4
  wires:
  "Kq3 "/1 -> Core controller: Torque,Power and Combined Torque/Power/12(K_q0r)
  Kq1/1 -> Core controller: Torque,Power and Combined Torque/Power/6(K_q0)
  Kt3/1 -> Core controller: Torque,Power and Combined Torque/Power/11(K_t0r)
  eps_c1/1 -> Core controller: Torque,Power and Combined Torque/Power/10(eps_c)
  Constant/1 -> Integrator/2
  Sum/1 -> Kp/1, Ki/1
  Sum1/1 -> Q_cn/1
  Integrator/1 -> Sum1/2
  Kp/1 -> Sum1/1
  Ki/1 -> Integrator/1
  n_r/1 -> Sum/1
  Core controller: Torque,Power and Combined Torque/Power/1(Qcq) -> Qcq/1
  Core controller: Torque,Power and Combined Torque/Power/2(Qcp) -> Qcp/1
  "Tr "/1 -> Core controller: Torque,Power and Combined Torque/Power/8(Tr)
  "n "/1 -> Core controller: Torque,Power and Combined Torque/Power/4(n), Sum/2
  Rho1/1 -> Core controller: Torque,Power and Combined Torque/Power/9(rho)
  D1/1 -> Core controller: Torque,Power and Combined Torque/Power/7(D)
  Ktf/1 -> Core controller: Torque,Power and Combined Torque/Power/5(K_t0)
  Core controller: Torque,Power and Combined Torque/Power/3(Qcc) -> Qcc/1
  Rcc/1 -> Core controller: Torque,Power and Combined Torque/Power/3(r_cc)
  Pcc/1 -> Core controller: Torque,Power and Combined Torque/Power/2(p_cc)
  Kcc/1 -> Core controller: Torque,Power and Combined Torque/Power/1(k_cc)

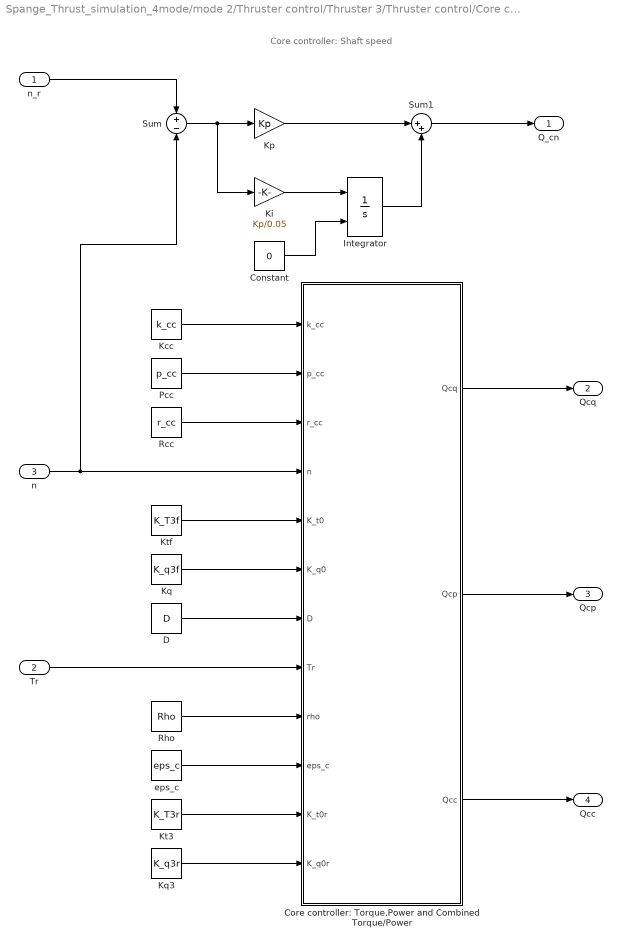
== system Spange_Thrust_simulation_4mode/mode 2/Thruster control/Thruster 3/Thruster control/Core controller ==
  note: Core controller: Shaft speed
  n_r : Inport
  "Tr " : Inport  Port=2
  "n " : Inport  Port=3
  Constant : Constant  Value=0
  Core controller: Torque,Power and Combined Torque/Power : MATLAB Function  TreatAsAtomicUnit=on
  D : Constant  Value=D
  Integrator : Integrator  ExternalReset=either
  Kcc : Constant  Value=k_cc
  Ki : Gain  Gain=Kp/0.05
  Kp : Gain  Gain=Kp
  Kq : Constant  Value=K_q3f
  "Kq3 " : Constant  Value=K_q3r
  Kt3 : Constant  Value=K_T3r
  Ktf : Constant  Value=K_T3f
  Pcc : Constant  Value=p_cc
  Rcc : Constant  Value=r_cc
  Rho : Constant  Value=Rho
  Sum : Sum  Inputs=+|-
  Sum1 : Sum  Inputs=|++
  eps_c : Constant  Value=eps_c
  Q_cn : Outport
  Qcq : Outport  Port=2
  Qcp : Outport  Port=3
  Qcc : Outport  Port=4
  wires:
  "Kq3 "/1 -> Core controller: Torque,Power and Combined Torque/Power/12(K_q0r)
  Kt3/1 -> Core controller: Torque,Power and Combined Torque/Power/11(K_t0r)
  eps_c/1 -> Core controller: Torque,Power and Combined Torque/Power/10(eps_c)
  Core controller: Torque,Power and Combined Torque/Power/1(Qcq) -> Qcq/1
  Core controller: Torque,Power and Combined Torque/Power/2(Qcp) -> Qcp/1
  "Tr "/1 -> Core controller: Torque,Power and Combined Torque/Power/8(Tr)
  "n "/1 -> Core controller: Torque,Power and Combined Torque/Power/4(n), Sum/2
  Rho/1 -> Core controller: Torque,Power and Combined Torque/Power/9(rho)
  Kq/1 -> Core controller: Torque,Power and Combined Torque/Power/6(K_q0)
  D/1 -> Core controller: Torque,Power and Combined Torque/Power/7(D)
  Ktf/1 -> Core controller: Torque,Power and Combined Torque/Power/5(K_t0)
  Core controller: Torque,Power and Combined Torque/Power/3(Qcc) -> Qcc/1
  Rcc/1 -> Core controller: Torque,Power and Combined Torque/Power/3(r_cc)
  Pcc/1 -> Core controller: Torque,Power and Combined Torque/Power/2(p_cc)
  Kcc/1 -> Core controller: Torque,Power and Combined Torque/Power/1(k_cc)
  Constant/1 -> Integrator/2
  Sum1/1 -> Q_cn/1
  Sum/1 -> Kp/1, Ki/1
  Integrator/1 -> Sum1/2
  Kp/1 -> Sum1/1
  Ki/1 -> Integrator/1
  n_r/1 -> Sum/1

== system Spange_Thrust_simulation_4mode/mode 3/Thruster control/Thruster 1/Thruster control/Core controller ==
  note: Core controller: Shaft speed
  n_r : Inport
  "Tr " : Inport  Port=2
  "n " : Inport  Port=3
  Constant : Constant  Value=0
  Core controller: Torque,Power and Combined Torque/Power : MATLAB Function  TreatAsAtomicUnit=on
  D1 : Constant  Value=D
  Integrator : Integrator  ExternalReset=either
  Kcc : Constant  Value=k_cc
  Ki : Gain  Gain=Kp/0.05
  Kp : Gain  Gain=Kp
  Kq1 : Constant  Value=K_q1f
  "Kq3 " : Constant  Value=K_q1r
  Kt3 : Constant  Value=K_T1r
  Ktf : Constant  Value=K_T1f
  Pcc : Constant  Value=p_cc
  Rcc : Constant  Value=r_cc
  Rho1 : Constant  Value=Rho
  Sum : Sum  Inputs=+|-
  Sum1 : Sum  Inputs=|++
  eps_c1 : Constant  Value=eps_c
  Q_cn : Outport
  Qcq : Outport  Port=2
  Qcp : Outport  Port=3
  Qcc : Outport  Port=4
  wires:
  "Kq3 "/1 -> Core controller: Torque,Power and Combined Torque/Power/12(K_q0r)
  Kq1/1 -> Core controller: Torque,Power and Combined Torque/Power/6(K_q0)
  Kt3/1 -> Core controller: Torque,Power and Combined Torque/Power/11(K_t0r)
  eps_c1/1 -> Core controller: Torque,Power and Combined Torque/Power/10(eps_c)
  Constant/1 -> Integrator/2
  Sum/1 -> Kp/1, Ki/1
  Sum1/1 -> Q_cn/1
  Integrator/1 -> Sum1/2
  Kp/1 -> Sum1/1
  Ki/1 -> Integrator/1
  n_r/1 -> Sum/1
  Core controller: Torque,Power and Combined Torque/Power/1(Qcq) -> Qcq/1
  Core controller: Torque,Power and Combined Torque/Power/2(Qcp) -> Qcp/1
  "Tr "/1 -> Core controller: Torque,Power and Combined Torque/Power/8(Tr)
  "n "/1 -> Core controller: Torque,Power and Combined Torque/Power/4(n), Sum/2
  Rho1/1 -> Core controller: Torque,Power and Combined Torque/Power/9(rho)
  D1/1 -> Core controller: Torque,Power and Combined Torque/Power/7(D)
  Ktf/1 -> Core controller: Torque,Power and Combined Torque/Power/5(K_t0)
  Core controller: Torque,Power and Combined Torque/Power/3(Qcc) -> Qcc/1
  Rcc/1 -> Core controller: Torque,Power and Combined Torque/Power/3(r_cc)
  Pcc/1 -> Core controller: Torque,Power and Combined Torque/Power/2(p_cc)
  Kcc/1 -> Core controller: Torque,Power and Combined Torque/Power/1(k_cc)

== system Spange_Thrust_simulation_4mode/mode 3/Thruster control/Thruster 2/Thruster control/Core controller ==
  note: Core controller: Shaft speed
  n_r : Inport
  "Tr " : Inport  Port=2
  "n " : Inport  Port=3
  Constant : Constant  Value=0
  Core controller: Torque,Power and Combined Torque/Power : MATLAB Function  TreatAsAtomicUnit=on
  D1 : Constant  Value=D
  Integrator : Integrator  ExternalReset=either
  Kcc : Constant  Value=k_cc
  Ki : Gain  Gain=Kp/0.05
  Kp : Gain  Gain=Kp
  Kq1 : Constant  Value=K_q2f
  "Kq3 " : Constant  Value=K_q2r
  Kt3 : Constant  Value=K_T2r
  Ktf : Constant  Value=K_T2f
  Pcc : Constant  Value=p_cc
  Rcc : Constant  Value=r_cc
  Rho1 : Constant  Value=Rho
  Sum : Sum  Inputs=+|-
  Sum1 : Sum  Inputs=|++
  eps_c1 : Constant  Value=eps_c
  Q_cn : Outport
  Qcq : Outport  Port=2
  Qcp : Outport  Port=3
  Qcc : Outport  Port=4
  wires:
  "Kq3 "/1 -> Core controller: Torque,Power and Combined Torque/Power/12(K_q0r)
  Kt3/1 -> Core controller: Torque,Power and Combined Torque/Power/11(K_t0r)
  eps_c1/1 -> Core controller: Torque,Power and Combined Torque/Power/10(eps_c)
  Core controller: Torque,Power and Combined Torque/Power/1(Qcq) -> Qcq/1
  Core controller: Torque,Power and Combined Torque/Power/2(Qcp) -> Qcp/1
  "Tr "/1 -> Core controller: Torque,Power and Combined Torque/Power/8(Tr)
  "n "/1 -> Sum/2, Core controller: Torque,Power and Combined Torque/Power/4(n)
  Rho1/1 -> Core controller: Torque,Power and Combined Torque/Power/9(rho)
  D1/1 -> Core controller: Torque,Power and Combined Torque/Power/7(D)
  Ktf/1 -> Core controller: Torque,Power and Combined Torque/Power/5(K_t0)
  Core controller: Torque,Power and Combined Torque/Power/3(Qcc) -> Qcc/1
  Rcc/1 -> Core controller: Torque,Power and Combined Torque/Power/3(r_cc)
  Pcc/1 -> Core controller: Torque,Power and Combined Torque/Power/2(p_cc)
  Kcc/1 -> Core controller: Torque,Power and Combined Torque/Power/1(k_cc)
  Constant/1 -> Integrator/2
  Sum1/1 -> Q_cn/1
  Sum/1 -> Kp/1, Ki/1
  Integrator/1 -> Sum1/2
  Kp/1 -> Sum1/1
  Ki/1 -> Integrator/1
  n_r/1 -> Sum/1
  Kq1/1 -> Core controller: Torque,Power and Combined Torque/Power/6(K_q0)

== system Spange_Thrust_simulation_4mode/mode 4/Thruster control/Thruster 1/Thruster control/Core controller ==
  note: Core controller: Shaft speed
  n_r : Inport
  "Tr " : Inport  Port=2
  "n " : Inport  Port=3
  Constant : Constant  Value=0
  Core controller: Torque,Power and Combined Torque/Power : MATLAB Function  TreatAsAtomicUnit=on
  D1 : Constant  Value=D
  Integrator : Integrator  ExternalReset=either
  Kcc : Constant  Value=k_cc
  Ki : Gain  Gain=Kp/0.05
  Kp : Gain  Gain=Kp
  Kq1 : Constant  Value=K_q1f
  "Kq3 " : Constant  Value=K_q1r
  Kt3 : Constant  Value=K_T1r
  Ktf : Constant  Value=K_T1f
  Pcc : Constant  Value=p_cc
  Rcc : Constant  Value=r_cc
  Rho1 : Constant  Value=Rho
  Sum : Sum  Inputs=+|-
  Sum1 : Sum  Inputs=|++
  eps_c1 : Constant  Value=eps_c
  Q_cn : Outport
  Qcq : Outport  Port=2
  Qcp : Outport  Port=3
  Qcc : Outport  Port=4
  wires:
  "Kq3 "/1 -> Core controller: Torque,Power and Combined Torque/Power/12(K_q0r)
  Kq1/1 -> Core controller: Torque,Power and Combined Torque/Power/6(K_q0)
  Kt3/1 -> Core controller: Torque,Power and Combined Torque/Power/11(K_t0r)
  eps_c1/1 -> Core controller: Torque,Power and Combined Torque/Power/10(eps_c)
  Constant/1 -> Integrator/2
  Sum/1 -> Kp/1, Ki/1
  Sum1/1 -> Q_cn/1
  Integrator/1 -> Sum1/2
  Kp/1 -> Sum1/1
  Ki/1 -> Integrator/1
  n_r/1 -> Sum/1
  Core controller: Torque,Power and Combined Torque/Power/1(Qcq) -> Qcq/1
  Core controller: Torque,Power and Combined Torque/Power/2(Qcp) -> Qcp/1
  "Tr "/1 -> Core controller: Torque,Power and Combined Torque/Power/8(Tr)
  "n "/1 -> Core controller: Torque,Power and Combined Torque/Power/4(n), Sum/2
  Rho1/1 -> Core controller: Torque,Power and Combined Torque/Power/9(rho)
  D1/1 -> Core controller: Torque,Power and Combined Torque/Power/7(D)
  Ktf/1 -> Core controller: Torque,Power and Combined Torque/Power/5(K_t0)
  Core controller: Torque,Power and Combined Torque/Power/3(Qcc) -> Qcc/1
  Rcc/1 -> Core controller: Torque,Power and Combined Torque/Power/3(r_cc)
  Pcc/1 -> Core controller: Torque,Power and Combined Torque/Power/2(p_cc)
  Kcc/1 -> Core controller: Torque,Power and Combined Torque/Power/1(k_cc)

== system Spange_Thrust_simulation_4mode/mode 4/Thruster control/Thruster 2/Thruster control/Core controller ==
  note: Core controller: Shaft speed
  n_r : Inport
  "Tr " : Inport  Port=2
  "n " : Inport  Port=3
  Constant : Constant  Value=0
  Core controller: Torque,Power and Combined Torque/Power : MATLAB Function  TreatAsAtomicUnit=on
  D1 : Constant  Value=D
  Integrator : Integrator  ExternalReset=either
  Kcc : Constant  Value=k_cc
  Ki : Gain  Gain=Kp/0.05
  Kp : Gain  Gain=Kp
  Kq1 : Constant  Value=K_q2f
  "Kq3 " : Constant  Value=K_q2r
  Kt3 : Constant  Value=K_T2r
  Ktf : Constant  Value=K_T2f
  Pcc : Constant  Value=p_cc
  Rcc : Constant  Value=r_cc
  Rho1 : Constant  Value=Rho
  Sum : Sum  Inputs=+|-
  Sum1 : Sum  Inputs=|++
  eps_c1 : Constant  Value=eps_c
  Q_cn : Outport
  Qcq : Outport  Port=2
  Qcp : Outport  Port=3
  Qcc : Outport  Port=4
  wires:
  "Kq3 "/1 -> Core controller: Torque,Power and Combined Torque/Power/12(K_q0r)
  Kt3/1 -> Core controller: Torque,Power and Combined Torque/Power/11(K_t0r)
  eps_c1/1 -> Core controller: Torque,Power and Combined Torque/Power/10(eps_c)
  Core controller: Torque,Power and Combined Torque/Power/1(Qcq) -> Qcq/1
  Core controller: Torque,Power and Combined Torque/Power/2(Qcp) -> Qcp/1
  "Tr "/1 -> Core controller: Torque,Power and Combined Torque/Power/8(Tr)
  "n "/1 -> Sum/2, Core controller: Torque,Power and Combined Torque/Power/4(n)
  Rho1/1 -> Core controller: Torque,Power and Combined Torque/Power/9(rho)
  D1/1 -> Core controller: Torque,Power and Combined Torque/Power/7(D)
  Ktf/1 -> Core controller: Torque,Power and Combined Torque/Power/5(K_t0)
  Core controller: Torque,Power and Combined Torque/Power/3(Qcc) -> Qcc/1
  Rcc/1 -> Core controller: Torque,Power and Combined Torque/Power/3(r_cc)
  Pcc/1 -> Core controller: Torque,Power and Combined Torque/Power/2(p_cc)
  Kcc/1 -> Core controller: Torque,Power and Combined Torque/Power/1(k_cc)
  Constant/1 -> Integrator/2
  Sum1/1 -> Q_cn/1
  Sum/1 -> Kp/1, Ki/1
  Integrator/1 -> Sum1/2
  Kp/1 -> Sum1/1
  Ki/1 -> Integrator/1
  n_r/1 -> Sum/1
  Kq1/1 -> Core controller: Torque,Power and Combined Torque/Power/6(K_q0)

== system Spange_Thrust_simulation_4mode/mode 4/Thruster control/Thruster 3/Thruster control/Core controller ==
  note: Core controller: Shaft speed
  n_r : Inport
  "Tr " : Inport  Port=2
  "n " : Inport  Port=3
  Constant : Constant  Value=0
  Core controller: Torque,Power and Combined Torque/Power : MATLAB Function  TreatAsAtomicUnit=on
  D : Constant  Value=D
  Integrator : Integrator  ExternalReset=either
  Kcc : Constant  Value=k_cc
  Ki : Gain  Gain=Kp/0.05
  Kp : Gain  Gain=Kp
  Kq : Constant  Value=K_q3f
  "Kq3 " : Constant  Value=K_q3r
  Kt3 : Constant  Value=K_T3r
  Ktf : Constant  Value=K_T3f
  Pcc : Constant  Value=p_cc
  Rcc : Constant  Value=r_cc
  Rho : Constant  Value=Rho
  Sum : Sum  Inputs=+|-
  Sum1 : Sum  Inputs=|++
  eps_c : Constant  Value=eps_c
  Q_cn : Outport
  Qcq : Outport  Port=2
  Qcp : Outport  Port=3
  Qcc : Outport  Port=4
  wires:
  "Kq3 "/1 -> Core controller: Torque,Power and Combined Torque/Power/12(K_q0r)
  Kt3/1 -> Core controller: Torque,Power and Combined Torque/Power/11(K_t0r)
  eps_c/1 -> Core controller: Torque,Power and Combined Torque/Power/10(eps_c)
  Core controller: Torque,Power and Combined Torque/Power/1(Qcq) -> Qcq/1
  Core controller: Torque,Power and Combined Torque/Power/2(Qcp) -> Qcp/1
  "Tr "/1 -> Core controller: Torque,Power and Combined Torque/Power/8(Tr)
  "n "/1 -> Core controller: Torque,Power and Combined Torque/Power/4(n), Sum/2
  Rho/1 -> Core controller: Torque,Power and Combined Torque/Power/9(rho)
  Kq/1 -> Core controller: Torque,Power and Combined Torque/Power/6(K_q0)
  D/1 -> Core controller: Torque,Power and Combined Torque/Power/7(D)
  Ktf/1 -> Core controller: Torque,Power and Combined Torque/Power/5(K_t0)
  Core controller: Torque,Power and Combined Torque/Power/3(Qcc) -> Qcc/1
  Rcc/1 -> Core controller: Torque,Power and Combined Torque/Power/3(r_cc)
  Pcc/1 -> Core controller: Torque,Power and Combined Torque/Power/2(p_cc)
  Kcc/1 -> Core controller: Torque,Power and Combined Torque/Power/1(k_cc)
  Constant/1 -> Integrator/2
  Sum1/1 -> Q_cn/1
  Sum/1 -> Kp/1, Ki/1
  Integrator/1 -> Sum1/2
  Kp/1 -> Sum1/1
  Ki/1 -> Integrator/1
  n_r/1 -> Sum/1

== matlab function Spange_Thrust_simulation_4mode/mode 4/T(F,alpha)/MATLAB Function ==
  data: thrust_actual input; actual_tau output; alpha_actual input; ThrusterPosX parameter; ThrusterPosY parameter
function actual_tau   = fcn(thrust_actual,alpha_actual,ThrusterPosX, ThrusterPosY)
%#codegen

Alpha_surge =[cosd(alpha_actual(1)) cosd(alpha_actual(2)) cosd(alpha_actual(3))];  
Alpha_sway = [sind(alpha_actual(1)) sind(alpha_actual(2)) sind(alpha_actual(3))];
Alpha_yaw = [sind(alpha_actual(1))*ThrusterPosX(1)-cosd(alpha_actual(1))*ThrusterPosY(1) sind(alpha_actual(2))*ThrusterPosX(2)-cosd(alpha_actual(2))*ThrusterPosY(2) ...
             sind(alpha_actual(3))*ThrusterPosX(3)-cosd(alpha_actual(3))*ThrusterPosY(3)];

actual_tau = [Alpha_surge;Alpha_sway;Alpha_yaw]*thrust_actual;

== matlab function Spange_Thrust_simulation_4mode/Mode enabler ==
  data: mode input; e1 output; e2 output; e3 output; e4 output
function [e1, e2, e3, e4] = fcn(mode)
%#codegen
e1 =0; e2 =0; e3 = 0; e4 = 0;
switch mode
    case 1,
        e1 = 1;
    case 2,
        e2 = 1;
    case 3,
        e3 = 1;
    case 4,
        e4 = 1;
end

== matlab function Spange_Thrust_simulation_4mode/mode 3/T(F,alpha)/MATLAB Function ==
  data: thrust_actual input; actual_tau output; alpha_actual input; PosX input; PosY input
function actual_tau   = fcn(thrust_actual,alpha_actual,PosX,PosY)
%#codegen

Alpha_surge =[cosd(alpha_actual(1)) cosd(alpha_actual(2))];  
Alpha_sway = [sind(alpha_actual(1)) sind(alpha_actual(2))];
Alpha_yaw = [sind(alpha_actual(1))*PosX(1)-cosd(alpha_actual(1))*PosY(1) sind(alpha_actual(2))*PosX(2)-cosd(alpha_actual(2))*PosY(2)];

actual_tau = [Alpha_surge;Alpha_sway;Alpha_yaw]*thrust_actual;

== matlab function Spange_Thrust_simulation_4mode/mode 3/Thrus & angle aloc/For Each Subsystem/Ensures fastest way is chosen ==
  data: desired input; psi_D output; actual input
function psi_D   = OptimalAngle(desired,actual)
%#codegen
psi_D = desired-actual;
if abs(psi_D) >= 360
    psi_D = rem(psi_D,360);
end

if abs(psi_D) >= 180
    psi_D = psi_D - sign(psi_D)*360;
end

== matlab function Spange_Thrust_simulation_4mode/mode 3/Thrus & angle aloc/For Each Subsystem/MATLAB Function ==
  data: angle input; y output
function y = rad2pipi(angle)
% RAD2PIPI Converts an angle in rad to the interval (-pi pi]
%          Should be applied to all heading errors in a feedback control system
%          in order to avoid discontinuities.
%
% Author:     Roger Skjetne
% Date:       2003-09-05
% Revisions:  2004-09-02 Thor I. Fossen - replaced input argument x with angle
%             2005-01-05 Thor I. Fossen - ouput argument is set to y and not angle
%             2005-04-13 Roger Skjetne  - changed the function s in order
%                                         to account for correct mapping to
%                                         (-pi pi].
%
% ________________________________________________________________
%
% MSS GNC is a Matlab toolbox for guidance, navigation and control.
% The toolbox is part of the Marine Systems Simulator (MSS).
%
% Copyright (C) 2008 Thor I. Fossen and Tristan Perez
% 
% This program is free software: you can redistribute it and/or modify
% it under the terms of the GNU General Public License as published by
% the Free Software Foundation, either version 3 of the License, or
% (at your option) any later version.
% 
% This program is distributed in the hope that it will be useful, but
% WITHOUT ANY WARRANTY; without even the implied warranty of
% MERCHANTABILITY or FITNESS FOR A PARTICULAR PURPOSE.  See the 
% GNU General Public License for more details.
% 
% You should have received a copy of the GNU General Public License
% along with this program.  If not, see <http://www.gnu.org/licenses/>.
% 
% E-mail: contact@marinecontrol.org
% URL:    <http://www.marinecontrol.org>


% convert angle in rad to the interval <-pi pi> 
r = rem(angle+sign(angle)*pi,2*pi);
s = sign(sign(angle) + 2*(sign(abs(rem(angle+pi,2*pi)/(2*pi)))-1));
% s = sign(angle);

y = r - s*pi;

== matlab function Spange_Thrust_simulation_4mode/mode 3/Thruster control/Thruster 1/Propeller Hydrodynamics/Actual Force and Torque ==
  data: Ta output; n input; Qa output; Kq input; Kt input; Ktr input; Kqr input; Rho input; D input; eps_c input; env input
function [Ta,Qa]= ActualForces(n,Kq,Kt,Ktr,Kqr,Rho,D,eps_c,env)
%#codegen
lambda_c = 0.5+0.5*tanh(eps_c*n/5); % Smooth switching between positive and negative thrust. 5 makes switch happen between -5 and 5
K_TC = Kt*lambda_c+(1-lambda_c)*Ktr;
K_QC = Kq*lambda_c+(1-lambda_c)*Kqr;

Ta = sign(n)*K_TC*Rho*(D^4)*n^2-env;
Qa = sign(n)*K_QC*Rho*(D^5)*n^2-env;
